simulink model "iqc_lib"  (Simulink 6.0)
settings: Solver=ode45  StartTime=0.0  StopTime=999999  MaxStep=10  RelTol=1e-3  AbsTol=1e-6
libraries: simulink x1
settings Model: Creator=user  LastModifiedBy=MD710
settings DataIOCC: LimitDataPoints=off  SaveOutput=off  SaveTime=off
settings OptimizationCC: BlockReduction=off  BooleanDataType=off  InlineInvariantSignals=off  InitFltsAndDblsToZero=off
settings DebuggingCC: SignalResolutionControl=UseLocalSettings  SolverPrmCheckMsg=none  MultiTaskDSMMsg=warning  MultiTaskCondExecSysMsg=none  FcnCallInpInsideContextMsg=Use local settings  StrictBusMsg=None  SFUnexpectedBacktrackingDiag=warning  SFNoUnconditionalDefaultTransitionDiag=warning
settings HardwareCC: TargetHWDeviceType=32-bit Generic
settings RTWCC: IncludeERTFirstTime=on
settings CodeAppCC: CustomSymbolStrType=$N$R$M

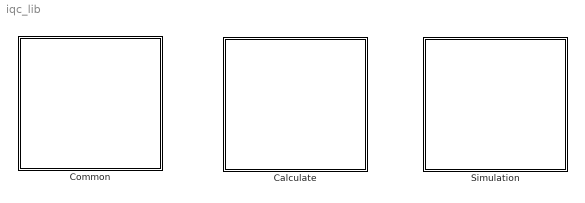
== system iqc_lib ==
  Calculate : Subsystem
      mask Display: disp('Calculate')
  Common : Subsystem
      mask Display: disp('Common')
  Simulation : Subsystem
      mask Display: disp('Simulation')

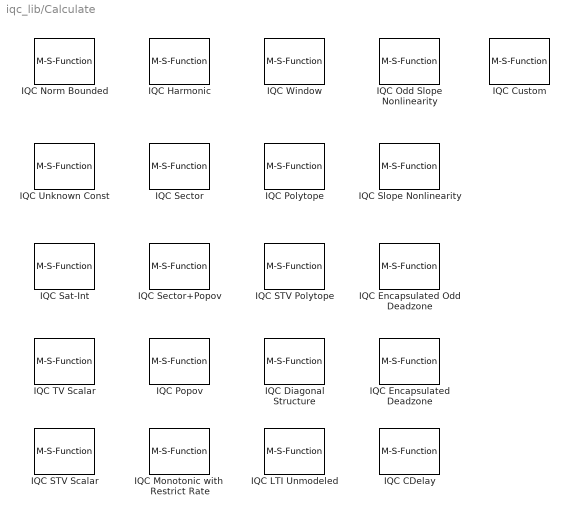
== system iqc_lib/Calculate ==
  IQC CDelay : M-S-Function  MFile=ext_iqc_cdelay  Parameters=max_tim,pole,out_var  mask(IQC cdelay(ver:0.1)){max_tim=1, pole=[], out_var=''}
      mask prompts: max_tim "Maximum Time Delay:(Default: 1)"; pole "Pole:(Default: [])"; out_var "Output Variable:(Default: empty)"
      mask help:
      | Example: [w,X,x]=iqc_cdelay(v,T,a)
      | Maximum Time Delay:
      |         T
      | Pole:
      |        [a]
      | Output Variable:
      |      {'X','x'}
      mask Help: eval('doc iqc_cdelay')
      mask Display: disp('\fontsize{16}e^{-ds}-1', 'texmode','on')
  IQC Custom : M-S-Function  MFile=ext_iqc_custom  Parameters=out_dim,list_iqc_rel  mask(IQC Custom(ver:0.1)){out_dim=-1, list_iqc_rel='out==iqc_popov_vect(in,0)|out==iqc_tvscalar(in,1)'}
      mask prompts: out_dim "Output Signal Dimensions:(Default: -1)"; list_iqc_rel "List of IQC Relationships:"
      mask Display: disp('Custom')
  IQC Diagonal Structure : M-S-Function  MFile=ext_iqc_diag  Parameters=out_var  mask(IQC Diagonal Structure(ver:0.1)){out_var=''}
      mask prompts: out_var "Output Variable:(Default: empty)"
      mask help:
      | Example: [w,X]=iqc_diag(v)
      | Output Variable:
      |             {'X'}
      mask Help: eval('doc iqc_diag')
      mask Display: plot(0,0,100,100,[20,7,7,20],[5,5,94,94],[22,33,11,22],[90,66,66,90],[43,55,32,43],[61,36,36,62],[62,63,62,61,62],[31,29,27,29,31],[71,72,71,70,71],[17,15,13,15,17],[78,90,90,79],[94,94,5,5])
  IQC Encapsulated Deadzone : M-S-Function  MFile=ext_iqc_dzn_e  Parameters=pole,def_num_h,slo_bou,out_var  mask(IQC Encapsulated Deadzone(ver:0.1)){pole=[1], def_num_h=0, slo_bou=1, out_var=''}
      mask prompts: pole "Pole:(Default: [1])"; def_num_h "Defines Number of Terms in Expansion for H:(Default: 0)"; slo_bou "Slope Bound for The Encapsulated Nonlinearity:(Default: 1)"; out_var "Output Variable:(Default: empty)"
      mask help:
      | Example: [w,h_0,H,F,x]=iqc_dzn_e(v,a,N,kdzn)
      | Pole:
      |       [a]
      | Defines Number of Terms in Expansion for H:
      |        N
      | Slope Bound for The Encapsulated Nonlinearity:
      |      kdzn
      | Output Variable:
      |    {'h_0','H','F','x'}
      mask Help: eval('doc iqc_dzn_e')
      mask Display: plot(0,0,100,100,[60,30,30,60,60],[90,90,60,60,90],[30,30,60,60,30],[40,10,10,40,40],[30,10,10,3,30],[25,25,76,76,76],[80,80,60],[72,25,25],[60,77],[76,76],[82,80,77,80,82,98],[76,72,76,80,76,76],[58,50,40,32],[88,76,76,63],[42,45,45,50],[15,17,34,36])
  IQC Encapsulated Odd Deadzone : M-S-Function  MFile=ext_iqc_dzn_e_odd  Parameters=pole,def_num_h,slo_bou,out_var  mask(IQC Encapsulated Odd Deadzone(ver:0.1)){pole=[1], def_num_h=0, slo_bou=1, out_var=''}
      mask prompts: pole "Pole:(Default: [1])"; def_num_h "Defines Number of Terms in Expansion for H:(Default: 0)"; slo_bou "Slope Bound for The Encapsulated Nonlinearity:(Default: 1)"; out_var "Output Variable:(Default: empty)"
      mask help:
      | Example: [w,h_0,H,F,xp,xm]=iqc_dzn_e_odd(v,a,N,kdzn)
      | Pole:
      |         [a]
      | Defines Number of Terms in Expansion for H:
      |          N
      | Slope Bound for The Encapsulated Nonlinearity:
      |         kdzn
      | Output Variable:
      |     {'h_0','H','F','xp','xm'}
      mask Help: eval('doc iqc_dzn_e_odd')
      mask Display: plot(0,0,100,100,[60,30,30,60,60],[90,90,60,60,90],[30,30,60,60,30],[40,10,10,40,40],[30,10,10,3,30],[25,25,76,76,76],[80,80,60],[72,25,25],[60,77],[76,76],[82,80,77,80,82,98],[76,72,76,80,76,76],[58,50,40,32],[88,76,76,63],[42,45,45,50],[15,17,34,36])
  IQC Harmonic : M-S-Function  MFile=ext_iqc_harmonic  Parameters=del_fre,pole,out_var  mask(IQC Harmonic(ver:0.1)){del_fre=1, pole=[1], out_var=''}
      mask prompts: del_fre "Delta Frequency:(Default: 1)"; pole "Pole:(Default: [1])"; out_var "Output Variable:(Default: empty)"
      mask help:
      | Example: [w,P,Q,X]=iqc_harmonic(v,w0,a)
      | Delta Frequency:
      |               w0
      | Pole:
      |               [a]
      | Output Variable:
      |               {'P','Q','X'}
      mask Help: eval('doc iqc_harmonic')
      mask Display: plot(1:0.1:15,cos(1:0.1:15))
  IQC LTI Unmodeled : M-S-Function  MFile=ext_iqc_ltiunmod  Parameters=pole,out_dim,upp_bou,out_var  mask(IQC LTI Unmodeled(ver:0.1)){pole=1, out_dim=-1, upp_bou=1, out_var=''}
      mask prompts: pole "Pole:(Default: [1])"; out_dim "The Dimension of The Output Signal:(Default: -1)"; upp_bou "Upper Bound of The H-inf norm of delta:(Default: 1)"; out_var "Output Variable:(Default: empty)"
      mask help:
      | Example: [w,X]=iqc_ltiunmod(v,a,n,g)
      | Pole:
      |      [a]
      | The Dimension of The Output Signal:
      |       n
      | Upper Bound of The H-inf norm of delta:
      |       g
      | Output Variable:
      |      {'X'}
      mask Help: eval('doc iqc_ltiunmod')
      mask Display:
      | disp('\fontsize{16}\Delta(S)', 'texmode','on');
      | % plot(0,0,100,100,[81,85,86,85,81],[19,34,44,56,72],[54,57,62,71,74,75,74,68,60,55,53,55,60,67,74],[32,27,25,25,28,34,41,48,51,53,59,66,69,69,66],[45,43,42,43,45],[20,37,46,57,72],[25,10,36,25],[71,24,24,72])
  IQC Monotonic with  Restrict Rate : M-S-Function  MFile=ext_iqc_monotonic  Parameters=pole,int_dd,ope,out_var  mask(IQC Monotonic with Restrict Rate(ver:0.1)){pole=[1], ope=0 (shut off the Popov's IQC), int_dd=1, out_var=''}
      mask prompts: pole "Pole:(Default: [1])"; ope "Operator:(Default: 0)"; int_dd "Interval of d(delta)/dt:(Default: 1)"; out_var "Output Variable:(Default: empty)"
      mask help:
      | Example: [w,xa,xb,xc,xd,xpop]=iqc_monotonic(v,a,op,k)
      | Pole:
      |          [a]
      | Operator:
      |          [op]
      | Interval of d(delta)/dt:
      |          [k]
      | Output Variable:
      |          {'xa','xb','xc','xd','xpop'}
      mask Help: eval('doc iqc_monotonic')
      mask StyleString: edit,popup(0 (shut off the Popov's IQC)|1 (turn on the Popov's IQC)),edit,edit
      mask Display: plot(0,0,100,100,[99,-0],[50,50],[50,50],[-0,100],[10,90],[0,100],[99,95,88,82,75,70,67,60,55,50],[76,76,75,74,72,70,68,62,56,50],[1,5,9,16,22,29,34,40,45,50],[20,21,22,24,26,29,32,38,44,50])
  IQC Norm Bounded : M-S-Function  MFile=ext_iqc_ltvnorm  Parameters=out_dim,max_amp,out_var  mask(IQC Norm Bounded(ver:0.1)){out_dim=1, max_amp=1, out_var=''}
      mask prompts: out_dim "The Dimension of the Output Signal:(Default: 1)"; max_amp "Maximal Amplification Ratio:(Default: 1)"; out_var "Output Variable:(Default: Empty)"
      mask help:
      | Example: [w,X]=iqc_ltvnorm(v,n,g)
      | The Dimemsion of the Output Signal:
      |            n
      | Maximal Amplification Ration:
      |            g
      | Output Variable:
      |            {'X'}
      mask Help: eval('doc iqc_ltvnorm')
      mask Display: disp('\fontsize{16}||\Delta|| < k', 'texmode','on')
  IQC Odd Slope Nonlinearity : M-S-Function  MFile=ext_iqc_slope_odd  Parameters=pole,len_def_h,low_bou,upp_bou,out_var  mask(IQC Odd Slope Nonlinearity(ver:0.1)){pole=[1], len_def_h=0, low_bou=0, upp_bou=1, out_var=''}
      mask prompts: pole "Pole:(Default: [1])"; len_def_h "Length of The Expansion that Defines H:(Default: 0)"; low_bou "Lower Bound on Slope:(Default: 0)"; upp_bou "Upper Bound on Slope:(Default: 1)"; out_var "Output Variable:(Default: empty)"
      mask help:
      | Example: [w,h0,H,xp,xm]=iqc_slope_odd(v,a,N,alpha,beta)
      | Pole:
      |          [a]
      | Length of The Expansion that Defines H:
      |           N
      | Lower Bound on Slope:
      |         alpha
      | Upper Bound on Slope:
      |         beta
      | Output Variable:
      |    {'h0','H','xp','xm'}
      mask Help: eval('doc iqc_slope_odd')
      mask Display: plot(0,0,100,100,[96,2],[50,50],[50,50],[95,4],[97,80,60,40,20,4],[90,90,71,30,10,10],[81,84,60,75,60],[72,71,71,99,71],[81,84],[69,71],[73,75],[97,99],[75,75,75],[96,99,99])
  IQC Polytope : M-S-Function  MFile=ext_iqc_polytope  Parameters=arr_pol,out_var  mask(IQC Polytope(ver:0.1)){arr_pol={''}, out_var=''}
      mask prompts: arr_pol "A Cell Array Containing The Vertices of The Polytope:"; out_var "Output Variable:(Default: empty)"
      mask help:
      | Example: [w,X,Y,Z]=iqc_polytope(v,C)
      | A Cell Array Containing The Vertices of The Polytope:
      |                    C
      | Output Variable:
      |              {'X','Y','Z'}
      mask Help: eval('doc iqc_polytope')
      mask Display: plot(0,0,100,100,[33,15,33,67,84,67,33],[80,50,20,20,50,80,80])
  IQC Popov : M-S-Function  MFile=ext_iqc_popov_vect  Parameters=sign_par,out_var  mask(IQC Popov(ver:0.1)){sign_par='0', out_var=''}
      mask prompts: sign_par "Sign of The Popov Parameter:(Default: '0')"; out_var "Output Variable:(Default: empty)"
      mask help:
      | Example: [w,Lambda]=iqc_popov_vect(v,'+')
      | Sign of The Popov Parameter:
      |                     '+'
      | Output Variable:
      |                  {'Lambda'}
      mask Help: eval('doc iqc_popov_vect')
      mask StyleString: popup('0'|'+'|'-'),edit
      mask Display: disp('Popov')
  IQC STV Polytope : M-S-Function  MFile=ext_iqc_polytope_stvp  Parameters=arr_del,arr_ddel,str_mat,out_var  mask(IQC STV Polytope(ver:0.1)){arr_del={''}, arr_ddel={''}, str_mat=[], out_var=''}
      mask prompts: arr_del "Cell Array for delta:"; arr_ddel "Cell Array for d(delta)/dt:"; str_mat "LMI-Lab Structure Matrix:"; out_var "Output Variable:(Default: empty)"
      mask help:
      | Example: [w,X,Y,Z,Lambda]=iqc_polytope_stvp(v,C1,C2,Lambdastruc);
      | Cell Array for delta:
      |              C1
      | Cell Array for d(delta)/dt
      |              C2
      | LMI-Lab Structure Matrix:
      |          Lambdastruc
      | Output Variable:
      |        {'X','Y','Z','Lambda'}
      mask Help: eval('doc iqc_polytope_stvp')
      mask Display: disp('STV\nPolytopic')
  IQC STV Scalar : M-S-Function  MFile=ext_iqc_slowtv  Parameters=upp_bou_dd,pole,upp_bou_d,out_var  mask(IQC STV Scalar(ver:0.1)){upp_bou_dd=1, pole=[1], upp_bou_d=1, out_var=''}
      mask prompts: upp_bou_dd "Upper Bound of The L-inf norm of d(delta)/dt:(Default: 1)"; pole "Pole:(Default [1])"; upp_bou_d "Upper Bound of The L-inf norm of delta:(Default: 1)"; out_var "Output Variable:(Default: empty)"
      mask help:
      | Example: [w,K1,M1,K2,M2]=iqc_slowtv(v,d,a,D)
      | Upper Bound of The L-inf norm of d(delta)/dt:
      |                   d
      | Pole:
      |                  [a]
      | Upper Bound of The L-inf norm of (delta):
      |                   D
      | Output Variable:
      |                  {'K1','M1','K2','M2'}
      mask Help: eval('doc iqc_slowtv')
      mask Display: disp('\fontsize{16}|D^\prime| < k', 'texmode','on')
  IQC Sat-Int : M-S-Function  MFile=ext_iqc_ratelimiter  Parameters=pole,k,out_var  mask(IQC Sat-Int(ver:0.1)){pole=[1,1], k=1, out_var=''}
      mask prompts: pole "Pole:(Default: [1,1])"; k "d(sat(0))/dt Value:(Default: 1)"; out_var "Output Variable:(Default: empty)"
      mask help:
      | Example: [w,M]=iqc_ratelimiter(v,a,k)
      | Pole:
      |     [a]
      | d(sat(0))/dt Value:
      |      k
      | Output Variable:
      |     {'M'}
      mask Help: eval('doc iqc_ratelimiter')
      mask Display: plot(0,0,100,100,[18,45,45,18,18],[60,60,26,26,60],[62,82,82,62,62],[60,60,26,26,60],[62,0],[44,44],[79,65],[44,44],[71,71],[46,57],[68,69,72,74,73,71,69,68,69,72,74],[31,29,29,31,34,35,36,38,40,40,39],[31,31],[26,60],[45,38,24],[55,55,33],[24,18],[33,33],[99,82],[44,44],[10,12,8,10,10,90,90],[44,51,51,44,80,80,44],[7,2],[55,55])
  IQC Sector : M-S-Function  MFile=ext_iqc_sector  Parameters=low_sec,upp_sec,out_var  mask(IQC Sector(ver:0.1)){low_sec=0, upp_sec=1, out_var=''}
      mask prompts: low_sec "Lower Sector Bound:(Default: 0)"; upp_sec "Upper Sector Bound:(Default: 1)"; out_var "Output Variable:(Default: empty)"
      mask help:
      | Example: [w,X]=iqc_sector(v,alpha,beta)
      | Lower Sector Bound:
      |              alpha
      | Upper Sector Bound:
      |              beta
      | Output Variable:
      |              {'X'}
      mask Help: eval('doc iqc_sector')
      mask Display: plot(0,0,100,100,[100,-0],[54,54],[50,50],[0,100],[66,32],[100,0],[-0,100],[37,71],[20,-0],[0,32],[33,13],[5,41],[40,28],[24,46],[47,42],[44,51],[65,57],[60,73],[78,63],[64,90],[95,77],[69,100],[91,85,82,78,77,75,74,66,61,56,54,50,48,45,43,42,40,38,35,31,27,24,21,17,14,11,10,8,7],[96,96,93,90,82,76,71,66,66,63,60,54,51,49,46,42,38,34,32,32,32,32,32,31,29,27,24,18,13])
  IQC Sector+Popov : M-S-Function  MFile=ext_iqc_popov  Parameters=low_sec,upp_sec,out_var  mask(IQC Sector+Popov(ver:0.1)){low_sec=0, upp_sec=1, out_var=''}
      mask prompts: low_sec "Low Sector Bound:(Default: 0)"; upp_sec "Upper Sector Bound:(Default: 1)"; out_var "Output Variable:(Default: empty)"
      mask help:
      | Example: [w,X,Y]=iqc_popov(v,alpha,beta)
      | Low Sector Bound:
      |                alpha
      | Upper Sector Bound:
      |                beta
      | Output Variable:
      |                {'X','Y'}
      mask Help: eval('doc iqc_popov')
      mask Display: plot(0,0,100,100,[100,-0],[54,54],[50,50],[0,100],[66,32],[100,0],[-0,100],[37,71],[20,-0],[0,32],[33,13],[5,41],[40,28],[24,46],[47,42],[44,51],[65,57],[60,73],[78,63],[64,90],[95,77],[69,100],[91,85,82,78,77,75,74,66,61,56,54,50,48,45,43,42,40,38,35,31,27,24,21,17,14,11,10,8,7],[96,96,93,90,82,76,71,66,66,63,60,54,51,49,46,42,38,34,32,32,32,32,32,31,29,27,24,18,13])
  IQC Slope Nonlinearity : M-S-Function  MFile=ext_iqc_slope  Parameters=pole,len_def_h,low_bou,upp_bou,out_var  mask(IQC Slope Nonlinearity(ver:0.1)){pole=[1], len_def_h=0, low_bou=0, upp_bou=1, out_var=''}
      mask prompts: pole "Pole:(Default: [1])"; len_def_h "Length of The Expansion that Defines H:(Default: 0)"; low_bou "Lower Bound on Slope:(Default: 0)"; upp_bou "Upper Bound on Slope:(Default: 1)"; out_var "Output Variable:(Default: empty)"
      mask help:
      | Example: [w,h0,H,x]=iqc_slope(v,a,N,alpha,beta)
      | Pole:
      |         [a]
      | Length of The Expansion that Defines H:
      |          N
      | Lower Bound on Slope:
      |        alpha
      | Upper Bound on Slope:
      |        beta
      | Output Variable:
      |    {'h0','H','x'}
      mask Help: eval('doc iqc_slope')
      mask Display: plot(0,0,100,100,[95,4],[50,50],[50,50],[95,5],[98,79,60,50,40,20,4],[90,90,80,50,40,30,30],[81,84,60,67,60],[82,80,80,100,80],[80,84],[78,80],[64,67],[98,100],[68,67,67,67,67],[96,100,100,100,100])
  IQC TV Scalar : M-S-Function  MFile=ext_iqc_tvscalar  Parameters=upp_bou,out_var  mask(IQC TV Scalar(ver:0.1)){upp_bou=1, out_var=''}
      mask prompts: upp_bou "Upper Bound of The L-inf norm of delta:(Default: 1)"; out_var "Output Variable:(Default: empty)"
      mask help:
      | Example: [w,X,Y]=iqc_tvscalar(v,D)
      | Upper Bound of The L-inf norm of delta:
      |         [D]
      | Output Variable:
      |         {'X','Y'}
      mask Help: eval('doc iqc_tvscalar')
      mask Display: disp('\fontsize{16}|D(t)| < k', 'texmode','on')
  IQC Unknown Const : M-S-Function  MFile=ext_iqc_ltigain  Parameters=pole,out_var  mask(IQC Unknown Const(ver:0.1)){pole=[1], out_var=''}
      mask prompts: pole "Pole:(Default: [1])"; out_var "Output Variable:(Default: Empty)"
      mask help:
      | Example: [w,P,Q,X,Y,Z]=iqc_ltigain(v,a);
      | Pole:
      |       [a]
      | Output Variable:
      |       {'P','Q','X','Y','Z'}
      mask Help: eval('doc iqc_ltigain')
      mask Display: disp('\fontsize{16}|d| < 1', 'texmode','on')
  IQC Window : M-S-Function  MFile=ext_iqc_window  Parameters=max_del,pole,out_var  mask(IQC Window(ver:0.1)){max_del=1, pole=[], out_var=''}
      mask prompts: max_del "Maximum Time Delay:(Default: 1)"; pole "Pole:(Default: [])"; out_var "Output Variable:(Default: empty)"
      mask help:
      | Example: [w,X,Y]=iqc_window(v,T,a)
      | Maximum Time Delay:
      |            T
      | Pole:
      |           [a]
      | Output Variable:
      |          {'X','Y'}
      mask Help: eval('doc iqc_window')
      mask Display: plot(0,0,100,100,[84,94,4],[27,25,25],[94,84],[25,22],[15,15],[5,97],[12,15],[86,97],[18,15],[86,97],[81,70,70,16,16,6],[26,26,72,72,26,26],[71,71,15],[26,73,73])

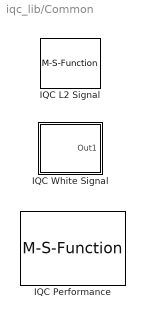
== system iqc_lib/Common ==
  IQC L2 Signal : M-S-Function  MFile=ext_iqc_L2signal  Parameters=sig_size,sam_time,sig_type,tru_time,sig_amp,sig_fre,user_cus  mask(IQC L2 signal(ver:0.1)){sig_size=1, sam_time=0, sig_type=Step, tru_time=10, sig_amp=1, sig_fre=1, user_cus='2*exp(3*t)'}
      mask prompts: sig_size "Signal Dimension:(Default: 1)"; sam_time "Sample Time:(Default: 0)"; sig_type "Signal Type:"; tru_time "Truncation Time:"; sig_amp "Maximum Amplitude:"; sig_fre "Frequency:"; user_cus "Custom:"
      mask help:
      | Important:
      | In IQC procedure step (as commond iqc_gain_tbx, the task is get
      | L2 gain value), regardless of the user to choose which option (ex sine...),
      | here regarded as generalized L2 signal.
      mask StyleString: edit,edit,popup(Step|Square wave|Sine wave|Custom|Random|External),edit,edit,edit,edit
      mask CallbackString: ||iqc_block_cho(gcb,'L2signal_type')||||
      mask TabNameString: Main,Main,Simulation,Simulation,Simulation,Simulation,Simulation
      mask Display: plot(0:0.1:10,[sin(0:0.1:6.2) zeros(1,38)])
  IQC Performance : M-S-Function  MFile=ext_iqc_performance  Parameters=imp_met,save_lin_com,isiqcbode,fre_ran,uselmitool,lmi_par  mask(IQC Performance(ver:0.1)){imp_met=Calculation and Simulation, save_lin_com=off, isiqcbode=off, fre_ran='', uselmitool=lmilab, lmi_par=''}
      mask prompts: imp_met "Implementation Methods"; save_lin_com "Save the Linear File and Command File"; isiqcbode "Display IQC Bode Figure"; fre_ran "Frequency Range:(Default: empty)"; uselmitool "LMI Tool:"; lmi_par "Parameter:(if empty use define)"
      mask help:
      | Important:
      | In IQC toolbox calculate step (as commond iqc_gain_tbx, the task is get
      | L2 gain value), regardless of the user to connect any signal input(Even if
      | not a signal), here regarded as generalized L2 signal.
      |
      | Example 1: setlmioptions('',[0 200 0 0 777])
      | the block parameter is
      | LMI Tool: lmilab
      | Parameter:
      |        [0 200 0 0 777]
      |
      | Example 2: setlmioptions('yalmip','solver','sdpt3','verbose',1)
      | the block parameter is
      | LMI Tool: yalmip
      | Parameter:
      |        {'solver',sdpt3','verbose',1}
      mask Help:
      | <a href="matlab:doc abst_init_iqc;">abst_init_iqc</a>
      | <a href="matlab:doc setlmioptions;">setlmioptions</a>
      | <a href="matlab:doc iqc_gain_tbx;">iqc_gain_tbx</a>
      mask StyleString: popup(Calculation and Simulation|Only Calculation|Only Simulation),checkbox,checkbox,edit,popup(lmilab|yalmip),edit
      mask CallbackString: iqc_block_cho(gcb,'performance_imp')||iqc_block_cho(gcb,'performance_bodefre')|||
      mask TabNameString: Main,Main,Main,Main,LMI,LMI
      mask Display: disp('In -> Out \n performance \n L2 gain:\n Unknown');
  IQC White Signal : Subsystem  mask(IQC White Signal(ver:0.1)){sig_size=1, sam_tim=0, ban_whi=10, pole=[1], out_var='', noi_pow=[0.1], seed=[23341]}
      mask prompts: sig_size "Signal Dimension:(Default: 1)"; sam_tim "Sample Time:(Default: 0)"; ban_whi "Bandwidth of White Signal:(Default: 10)"; pole "Pole:(Default: [1])"; out_var "Output Variable:(Default: empty)"; noi_pow "Noise Power:(Default: [0.1])"; seed "Seed:(Default: [23341])"
      mask help:
      | Example: [f,Y,Z]=iqc_white(n,b,a)
      | Bandwidth of White Signal:
      |           b
      | Pole:
      |           a
      | Output Variable:
      |    {'Y','Z'}
      mask init:
      | if any(noi_pow < 0),
      | 	error('The ''Noise power'' must be positive. '),
      | end;
      | if any(sam_tim==-1), 
      | 	error('You should explicitly specify the sample time of the source block. '), 
      | end
      | 
      | r = [0.4326
      |    -1.6656
      |     0.1253
      |     0.2877
      |    -1.1465
      |     1.1909
      |     -1.1892
      |    0.0376
      |     -0.3273
      |     0.1746
      |    -0.1867
      |     0.7258]';
      | t =[1:13;1:13]; 
      | r2 = [r(1),r;r,r(12)];
      mask Help: eval('doc iqc_white')
      mask TabNameString: Main,Main,Calculation,Calculation,Calculation,Simulation,Simulation
      mask Display: plot(t(:),r2(:))

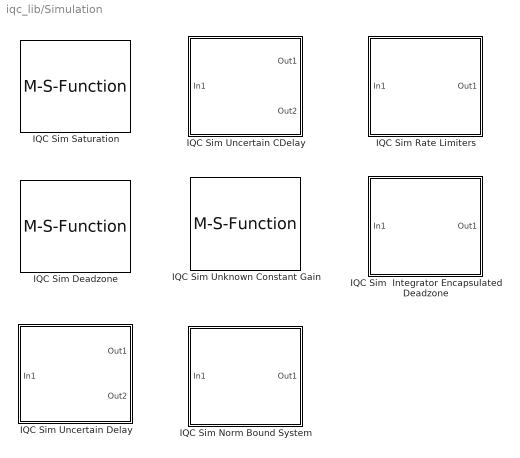
== system iqc_lib/Simulation ==
  IQC Sim Norm Bound System : Subsystem  mask(IQC Sim Norm Bound System(ver:0.1)){sou_sys=Random, num_inp=1, num_out=1, num_sta=1, upp_bou=1, sam_tim=0, cus='1/(s+1)', var_nam='', iqc1=on, iqc1_pole=[1], iqc1_out='', iqc2=off, lis_rel='', swsystemtype=0, A=0, B=0, C=0, D=0, newsam_tim=0}
      mask prompts: sou_sys "Source of the system:(Default: Random)"; num_inp "The Number of Input:(Default: 1)"; num_out "The Number of Output:(Default: 1)"; num_sta "The Number of States:(Default: 1)"; upp_bou "Upper Bound of the Hinf-Norm:(default: 1)"; sam_tim "Sample Time:(Default: 0)"; cus "Custom: (Default: '1/(s+1)' or '1/(z+0.5)')"; var_nam "Variable Name:(Default: empty)"; iqc1 "iqc_ltiunmod(Input,Pole,Number Output,Upper Bound)"; iqc1_pole "Pole:(Default: [1])"; iqc1_out "Output Variable:(Default: empty)"; iqc2 "Custom IQC"; lis_rel "List of IQC Relationships:"
      mask init:
      | swsystemtype=1;
      | A=randn(num_sta);
      | B=randn(num_sta,num_inp);
      | C=randn(num_out,num_sta);
      | D=randn(num_out,num_inp);
      | switch sou_sys
      |     case 1
      |         if sam_tim==0
      |             newsam_tim=1;
      |             A=A-(1+max(real(eig(A))))*eye(num_sta);
      |             G=ss(A,B,C,D);
      |             normG=norm(G,inf);
      |             G=G*upp_bou*rand/normG;
      |         elseif sam_tim>0
      |             newsam_tim=sam_tim;
      |             swsystemtype=2;
      |             A=A-(1+max(real(eig(A))))*eye(num_sta);
      |             G=ss(A,B,C,D);
      |             normG=norm(G,inf);
      |             G=G*upp_bou*rand/normG;
      |             G=c2d(G,sam_tim);
      |         else
      |             error(['sampletime set error'])
      |         end
      |     case 2
      |         s=tf('s');
      |         newsam_tim=1;
      |         if sam_tim>0
      |             newsam_tim=sam_tim;
      |             swsystemtype=2;
      |             z=tf('z',sam_tim);
      |         end
      |         if ischar(cus)
      |             eval(['G=ss(',cus,');']);
      |         else
      |             G=ss(cus);
      |         end
      | end
      | A=G.a;
      | B=G.b;
      | C=G.c;
      | D=G.d;
      mask Help: <a href="matlab:doc iqc_ltiunmod;">iqc_ltiunmod</a>
      mask StyleString: popup(Random|Custom),edit,edit,edit,edit,edit,edit,edit,checkbox,edit,edit,checkbox,edit,edit,edit,edit,edit,edit,edit
      mask CallbackString: iqc_block_cho(gcb,'sim_normboundsys_sou')||||||||iqc_block_cho(gcb,'sim_normboundsys_iqc1')|||iqc_block_cho(gcb,'sim_normboundsys_iqc2')|||||||
      mask TabNameString: Simulation,Simulation,Simulation,Simulation,Simulation,Simulation,Simulation,Simulation,Calculation,Calculation,Calculation,Calculation,Calculation,Simulation,Simulation,Simulation,Simulation,Simulation,Simulation
      mask Display: disp('\fontsize{14}||\Delta|| < k', 'texmode','on')
  IQC Sim Uncertain CDelay : Subsystem  mask(IQC Sim Uncertain CDelay(ver:0.1)){sou_del=Random, max_del=1, num_ran=1, cus=[0], iqc1=on, iqc1_pole=[], iqc1_out='', iqc2=off, lis_rel='', delay_time=0}
      mask prompts: sou_del "Source of the delay:(Default: Random)"; max_del "Maximum Delay:"; num_ran "The Number of Random:(1 or input_dim)"; cus "Custom:"; iqc1 "iqc_cdelay(Input,Maximum Delay,Pole)"; iqc1_pole "Pole:(Default: [])"; iqc1_out "Output Variable:(Default: empty)"; iqc2 "Custom IQC"; lis_rel "List of IQC Relationships:"
      mask init:
      | switch sou_del
      |     case 1
      |         delay_time=max_del*rand(1,num_ran);
      |     case 2
      |         delay_time=reshape(cus,1,length(cus));
      | end
      | % fprintf('The Random Delay Time: %4.3f \n',delay_time);
      mask Help: <a href="matlab:doc iqc_cdelay;">iqc_cdelay</a>
      mask StyleString: popup(Random|Custom),edit,edit,edit,checkbox,edit,edit,checkbox,edit,edit
      mask CallbackString: iqc_block_cho(gcb,'sim_uncertaincdelay_sou')||||iqc_block_cho(gcb,'sim_uncertaincdelay_iqc1')|||iqc_block_cho(gcb,'sim_uncertaincdelay_iqc2')||
      mask TabNameString: Simulation,Simulation,Simulation,Simulation,Calculation,Calculation,Calculation,Calculation,Calculation,Simulation
      mask Display:
      | disp('\fontsize{14}exp(-T*s)-1', 'texmode','on')
      | port_label('input',1,'in');
      | port_label('output',1,'out');
      | port_label('output',2,'T');
  IQC Sim Uncertain Delay : Subsystem  mask(IQC Sim Uncertain Delay(ver:0.1)){sou_del=Custom, max_del=1, num_ran=1, cus=[0.5], iqc1=on, iqc1_pole=[], iqc1_out='', iqc2=off, iqc2_pole=[], iqc2_out='', iqc3=off, lis_rel='', delay_time=0}
      mask prompts: sou_del "Source of the delay:(Default: Random)"; max_del "Maximum Delay:"; num_ran "The Number of Random:(1 or input_dim)"; cus "Custom:"; iqc1 "iqc_delay(Input,Maximum Delay,Pole)"; iqc1_pole "Pole:(Default: [])"; iqc1_out "Output Variable:(Default: empty)"; iqc2 "iqc_delay1(Input,Maximum Delay,Pole)"; iqc2_pole "Pole:(Default: [])"; iqc2_out "Output Variable:(Default: empty)"; iqc3 "Custom IQC"; lis_rel "List of IQC Relationships:"
      mask init:
      | switch sou_del
      |     case 1
      |         delay_time=max_del*rand(1,num_ran);
      |     case 2
      |         delay_time=reshape(cus,1,length(cus));
      | end
      | % fprintf('The Random Delay Time: %4.3f \n',delay_time);
      mask Help:
      | <a href="matlab:doc iqc_delay;">iqc_delay</a>
      | <a href="matlab:doc iqc_delay1;">iqc_delay1</a>
      mask StyleString: popup(Random|Custom),edit,edit,edit,checkbox,edit,edit,checkbox,edit,edit,checkbox,edit,edit
      mask CallbackString: iqc_block_cho(gcb,'sim_uncertaindelay_sou')||||iqc_block_cho(gcb,'sim_uncertaindelay_iqc1')|||iqc_block_cho(gcb,'sim_uncertaindelay_iqc2')|||iqc_block_cho(gcb,'sim_uncertaindelay_iqc3')||
      mask TabNameString: Simulation,Simulation,Simulation,Simulation,Calculation,Calculation,Calculation,Calculation,Calculation,Calculation,Calculation,Calculation,Simulation
      mask Display:
      | disp('\fontsize{14}exp(-T*s)', 'texmode','on')
      | port_label('input',1,'in');
      | port_label('output',1,'out');
      | port_label('output',2,'T');
  IQC Sim Unknown Constant Gain : M-S-Function  MFile=ext_sim_unknown_gain  Parameters=sou_con,num_ran,cus,iqc1,iqc1_pole,iqc1_out,iqc2,iqc2_out,iqc3,iqc3_out,iqc4,lis_rel,rand_cons  mask(IQC Sim Unknown Constant Gain(ver:0.1)){sou_con=Random, num_ran=1, cus=[0], iqc1=on, iqc1_pole=[1], iqc1_out='', iqc2=off, iqc2_out='', iqc3=off, iqc3_out='', iqc4=off, lis_rel='', rand_cons=0}
      mask prompts: sou_con "Source of The Constant Gain:(Default: Random)"; num_ran "The Number of Random:(1 or input_dim)"; cus "Custom:"; iqc1 "iqc_ltigain(Input,Pole)"; iqc1_pole "Pole:(Default: [1])"; iqc1_out "Output Variable:(Default: empty)"; iqc2 "iqc_ltvnorm(Input,length(Input),1)"; iqc2_out "Output Variable:(Default: empty)"; iqc3 "iqc_tvscalar(Input,1)"; iqc3_out "Output Variable:(Default: empty)"; iqc4 "Custom IQC"; lis_rel "List of IQC Relationships:"
      mask init:
      | switch sou_con
      |     case 1
      |         rand_cons=rand(1,num_ran);
      |     case 2
      |         if any(abs(cus)>1)
      |             error('the maximum random constant is 1')
      |         else
      |             rand_cons=reshape(cus,1,length(cus));
      |         end
      | end
      mask Help:
      | <a href="matlab:doc iqc_ltigain;">iqc_ltigain</a>
      | <a href="matlab:doc iqc_ltvnorm;">iqc_ltvnorm</a>
      | <a href="matlab:doc iqc_tvscalar;">iqc_tvscalar</a>
      mask StyleString: popup(Random|Custom),edit,edit,checkbox,edit,edit,checkbox,edit,checkbox,edit,checkbox,edit,edit
      mask CallbackString: iqc_block_cho(gcb,'sim_constantgain_sou')|||iqc_block_cho(gcb,'sim_constantgain_iqc1')|||iqc_block_cho(gcb,'sim_constantgain_iqc2')||iqc_block_cho(gcb,'sim_constantgain_iqc3')||iqc_block_cho(gcb,'sim_constantgain_iqc4')||
      mask TabNameString: Simulation,Simulation,Simulation,Calculation,Calculation,Calculation,Calculation,Calculation,Calculation,Calculation,Calculation,Calculation,Simulation
      mask Display:
      | disp('\fontsize{14}|d| < 1', 'texmode','on');
      | port_label('input',1,'in');
      | port_label('output',1,'out');
      | port_label('output',2,'|d|');
  IQC Sim  Integrator Encapsulated Deadzone : Subsystem  mask(IQC Sim Integrator Encapsulated Deadzone(ver:0.1)){sta_dea=-1, end_dea=1, slo=1, iqc1=on, iqc1_pole=[1], iqc1_def_num_h=0, iqc1_out='', iqc2=off, iqc2_pole=[1], iqc2_def_num_h=0, iqc2_out='', iqc3=off, lis_rel=''}
      mask prompts: sta_dea "Start of Deadzone:"; end_dea "End of Deadzone:"; slo "Slope:"; iqc1 "iqc_dzn_e(Input,Pole,N,Slope)"; iqc1_pole "Pole:(Default: [1])"; iqc1_def_num_h "Defines Number of Terms in Expansion for H:(Default: 0)"; iqc1_out "Output Variable:(Default: empty)"; iqc2 "iqc_dzn_e_odd(Input,Pole,N,Slope)"; iqc2_pole "Pole:(Default: [1])"; iqc2_def_num_h "Defines Number of Terms in Expansion for H:(Default: 0)"; iqc2_out "Output Variable:(Default: empty)"; iqc3 "Custom IQC"; lis_rel "List of IQC Relationships:"
      mask Help:
      | <a href="matlab:doc iqc_dzn_e;">iqc_dzn_e</a>
      | <a href="matlab:doc iqc_dzn_e_odd;">iqc_dzn_e_odd</a>
      mask CallbackString: |||iqc_block_cho(gcb,'sim_intencdeadzone_iqc1')||||iqc_block_cho(gcb,'sim_intencdeadzone_iqc2')||||iqc_block_cho(gcb,'sim_intencdeadzone_iqc3')|
      mask TabNameString: Simulation,Simulation,Simulation,Calculation,Calculation,Calculation,Calculation,Calculation,Calculation,Calculation,Calculation,Calculation,Calculation
      mask Display: plot(0,0,100,100,[60,30,30,60,60],[90,90,60,60,90],[30,30,60,60,30],[40,10,10,40,40],[30,10,10,3,30],[25,25,76,76,76],[80,80,60],[72,25,25],[60,77],[76,76],[82,80,77,80,82,98],[76,72,76,80,76,76],[58,50,40,32],[88,76,76,63],[42,45,45,50],[15,17,34,36])
  IQC Sim Deadzone : M-S-Function  MFile=ext_sim_deadzone  Parameters=sta_dea,end_dea,sam_tim,iqc1,iqc1_pole,iqc1_ope,iqc1_out,iqc2,iqc2_out,iqc3,iqc3_out,iqc4,iqc4_sign,iqc4_out,iqc5,lis_rel  mask(IQC Sim Deadzone(ver:0.2)){sta_dea=-1, end_dea=1, sam_tim=0, iqc1=on, iqc1_pole=[1], iqc1_ope=0 (shut off the Popov's IQC), iqc1_out='', iqc2=off, iqc2_out='', iqc3=off, iqc3_out='', iqc4=off, iqc4_sign='0', iqc4_out='', iqc5=off, lis_rel=''}
      mask prompts: sta_dea "Start of Deadzone:"; end_dea "End of Deadzone:"; sam_tim "Sample Time:"; iqc1 "iqc_monotonic(Input,Pole,Operator,1) (only for scalar input)"; iqc1_pole "Pole:(Default:[1])"; iqc1_ope "Operator:(Default: 0)"; iqc1_out "Output Variable:(Default: empty)"; iqc2 "iqc_sector(Input,0,1) (only for scalar input)"; iqc2_out "Output Variable:(Default: empty)"; iqc3 "iqc_popov(Input,0,1) (only for scalar input)"; iqc3_out "Output Variable:(Default: empty)"; iqc4 "iqc_popov_vect(Input,Sign)"; iqc4_sign "Sign:(Default: '0')"; iqc4_out "Output Variable:(Default: empty)"; iqc5 "Custom IQC"; lis_rel "List of IQC Relationships:"
      mask Help:
      | <a href="matlab:doc iqc_monotonic;">iqc_monotonic</a>
      | <a href="matlab:doc iqc_sector;">iqc_sector</a>
      | <a href="matlab:doc iqc_popov;">iqc_popov</a>
      | <a href="matlab:doc iqc_popov_vect;">iqc_popov_vect</a>
      mask StyleString: edit,edit,edit,checkbox,edit,popup(0 (shut off the Popov's IQC)|1 (turn on the Popov's IQC)),edit,checkbox,edit,checkbox,edit,checkbox,popup('0'|'+'|'-'),edit,checkbox,edit
      mask CallbackString: |||iqc_block_cho(gcb,'sim_deadzone_iqc1')||||iqc_block_cho(gcb,'sim_deadzone_iqc2')||iqc_block_cho(gcb,'sim_deadzone_iqc3')||iqc_block_cho(gcb,'sim_deadzone_iqc4')|||iqc_block_cho(gcb,'sim_deadzone_iqc5')|
      mask TabNameString: Simulation,Simulation,Simulation,Calculation,Calculation,Calculation,Calculation,Calculation,Calculation,Calculation,Calculation,Calculation,Calculation,Calculation,Calculation,Calculation
      mask Display:
      | x=-5:5;
      | for i=1:11
      |     if x(i)>=-2 && x(i)<=2
      |         y(i)=0;
      |     elseif x(i)<-2
      |         y(i)=x(i)+2;
      |     elseif x(i)>2
      |         y(i)=x(i)-2;
      |     end
      | end
      | x1=zeros(1,11);
      | y1=-5:1:5;
      | y2=zeros(1,11);
      | plot(x,y);
      | plot(x1,y1);
      | plot(x,y2);
  IQC Sim Rate Limiters : Subsystem  mask(IQC Sim Rate Limiters(ver:0.1)){upp_lim=1, low_lim=-1, d_sat=1, firstpole=1, iqc1=on, iqc1_pole=[1], iqc1_out='', iqc2=off, lis_rel=''}
      mask prompts: upp_lim "Upper Limit of Saturation:"; low_lim "Lower Limit of Saturation:"; d_sat "Slope of Saturation:(Default: 1)"; firstpole "(s+Pole1) ~ the Pole1:(Default: 1)"; iqc1 "iqc_ratelimiter(Input,[Pole1 Pole],Slope)  (only for scalar input)"; iqc1_pole "Pole:(Default: [1])"; iqc1_out "Output Variable:(Default: empty)"; iqc2 "Custom IQC"; lis_rel "List of IQC Relationships:"
      mask init:
      | if length(firstpole)>1
      |     error('the Pole1 only scalar')
      | end
      | if length(d_sat)>1
      |     error('d(Sat(0))/dt only scalar')
      | end
      mask Help: <a href="matlab:doc iqc_ratelimiter;">iqc_ratelimiter</a>
      mask CallbackString: ||||iqc_block_cho(gcb,'sim_ratelim_iqc1')|||iqc_block_cho(gcb,'sim_ratelim_iqc2')|
      mask TabNameString: Simulation,Simulation,Simulation,Simulation,Calculation,Calculation,Calculation,Calculation,Calculation
      mask Display: plot(0,0,100,100,[18,45,45,18,18],[60,60,26,26,60],[62,82,82,62,62],[60,60,26,26,60],[62,0],[44,44],[79,65],[44,44],[71,71],[46,57],[68,69,72,74,73,71,69,68,69,72,74],[31,29,29,31,34,35,36,38,40,40,39],[31,31],[26,60],[45,38,24],[55,55,33],[24,18],[33,33],[99,82],[44,44],[10,12,8,10,10,90,90],[44,51,51,44,80,80,44],[7,2],[55,55])
  IQC Sim Saturation : M-S-Function  MFile=ext_sim_saturation  Parameters=upp_lim,low_lim,sam_tim,iqc1,iqc1_pole,iqc1_ope,iqc1_out,iqc2,iqc2_out,iqc3,iqc3_out,iqc4,iqc4_sign,iqc4_out,iqc5,lis_rel  mask(IQC Sim Saturation(ver:0.1)){upp_lim=1, low_lim=-1, sam_tim=0, iqc1=on, iqc1_pole=[1], iqc1_ope=0 (shut off the Popov's IQC), iqc1_out='', iqc2=off, iqc2_out='', iqc3=off, iqc3_out='', iqc4=off, iqc4_sign='0', iqc4_out='', iqc5=off, lis_rel=''}
      mask prompts: upp_lim "Upper Limit:"; low_lim "Lower Limit:"; sam_tim "Sample Time:(Default: 0)"; iqc1 "iqc_monotonic(Input,Pole,Operator,1) (only for scalar input)"; iqc1_pole "Pole:(Default:[1])"; iqc1_ope "Operator:(Default: 0)"; iqc1_out "Output Variable:(Default: empty)"; iqc2 "iqc_sector(Input,0,1) (only for scalar input)"; iqc2_out "Output Variable:(Default: empty)"; iqc3 "iqc_popov(Input,0,1) (only for scalar input)"; iqc3_out "Output Variable:(Default: empty)"; iqc4 "iqc_popov_vect(Input,Sign)"; iqc4_sign "Sign:(Default: '0')"; iqc4_out "Output Variable:(Default: empty)"; iqc5 "Custom IQC"; lis_rel "List of IQC Relationships:"
      mask Help:
      | <a href="matlab:doc iqc_monotonic;">iqc_monotonic</a>
      | <a href="matlab:doc iqc_sector;">iqc_sector</a>
      | <a href="matlab:doc iqc_popov;">iqc_popov</a>
      | <a href="matlab:doc iqc_popov_vect;">iqc_popov_vect</a>
      mask StyleString: edit,edit,edit,checkbox,edit,popup(0 (shut off the Popov's IQC)|1 (turn on ther Popov's IQC)),edit,checkbox,edit,checkbox,edit,checkbox,popup('0'|'+'|'-'),edit,checkbox,edit
      mask CallbackString: |||iqc_block_cho(gcb,'sim_saturation_iqc1')||||iqc_block_cho(gcb,'sim_saturation_iqc2')||iqc_block_cho(gcb,'sim_saturation_iqc3')||iqc_block_cho(gcb,'sim_saturation_iqc4')|||iqc_block_cho(gcb,'sim_saturation_iqc5')|
      mask TabNameString: Simulation,Simulation,Simulation,Calculation,Calculation,Calculation,Calculation,Calculation,Calculation,Calculation,Calculation,Calculation,Calculation,Calculation,Calculation,Calculation
      mask Display:
      | x=-10:10;
      | for i=1:21;
      |     if x(i)>=-3 && x(i)<=3;
      |         y(i)=x(i);
      |     elseif x(i)<-3;
      |         y(i)=-3;
      |     elseif x(i)>3;
      |         y(i)=3;
      |     end
      | end
      | x1=zeros(1,11);
      | y1=-5:1:5;
      | y2=zeros(1,21);
      | plot(x,y);
      | plot(x1,y1);
      | plot(x,y2);

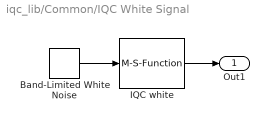
== system iqc_lib/Common/IQC White Signal ==
  Band-Limited White Noise : simulink/Sources/Band-Limited White Noise  Cov=noi_pow  Ts=sam_tim+0.01  seed=seed
  IQC white : M-S-Function  MFile=ext_iqc_white  Parameters=sig_size,ban_whi,pole,out_var,sam_tim
      mask Display: disp('IQC white \n S-function')
  Out1 : Outport
  wires:
  IQC white/1 -> Out1/1
  Band-Limited White Noise/1 -> IQC white/1

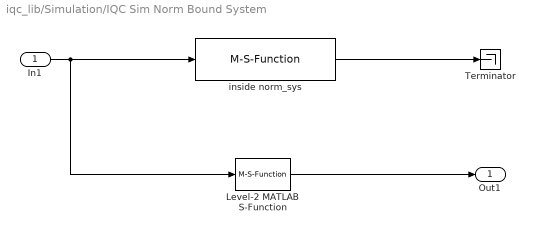
== system iqc_lib/Simulation/IQC Sim Norm Bound System ==
  In1 : Inport
  Level-2 MATLAB S-Function : M-S-Function  MFile=IQCSimSystem  Parameters=A,B,C,D,sam_tim
  Terminator : Terminator
  inside norm_sys : M-S-Function  MFile=ext_sim_normboundsystem  Parameters=sou_sys,num_inp,num_out,num_sta,upp_bou,sam_tim,cus,var_nam,iqc1,iqc1_pole,iqc1_out,iqc2,lis_rel,swsystemtype,A,B,C,D,
  Out1 : Outport
  wires:
  inside norm_sys/1 -> Terminator/1
  In1/1 -> Level-2 MATLAB S-Function/1, inside norm_sys/1
  Level-2 MATLAB S-Function/1 -> Out1/1

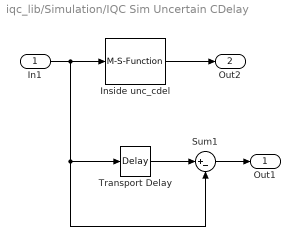
== system iqc_lib/Simulation/IQC Sim Uncertain CDelay ==
  In1 : Inport
  Inside unc_cdel : M-S-Function  MFile=ext_sim_uncertain_cdelay  Parameters=sou_del,max_del,num_ran,cus,iqc1,iqc1_pole,iqc1_out,iqc2,lis_rel,delay_time
  Sum1 : Sum  Inputs=|+-
  Transport Delay : TransportDelay  DelayTime=delay_time
  Out1 : Outport
  Out2 : Outport  Port=2
  wires:
  Inside unc_cdel/1 -> Out2/1
  Transport Delay/1 -> Sum1/1
  In1/1 -> Inside unc_cdel/1, Transport Delay/1, Sum1/2
  Sum1/1 -> Out1/1

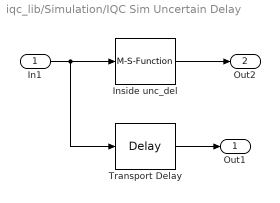
== system iqc_lib/Simulation/IQC Sim Uncertain Delay ==
  In1 : Inport
  Inside unc_del : M-S-Function  MFile=ext_sim_uncertain_delay  Parameters=sou_del,max_del,num_ran,cus,iqc1,iqc1_pole,iqc1_out,iqc2,iqc2_pole,iqc2_out,iqc3,lis_rel,delay_time
  Transport Delay : TransportDelay  DelayTime=delay_time
  Out1 : Outport
  Out2 : Outport  Port=2
  wires:
  In1/1 -> Inside unc_del/1, Transport Delay/1
  Transport Delay/1 -> Out1/1
  Inside unc_del/1 -> Out2/1

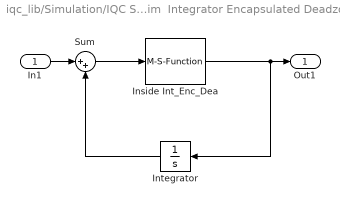
== system iqc_lib/Simulation/IQC Sim  Integrator Encapsulated Deadzone ==
  In1 : Inport
  Inside Int_Enc_Dea : M-S-Function  MFile=ext_sim_intenc_deadzone  Parameters=sta_dea,end_dea,slo,iqc1,iqc1_pole,iqc1_def_num_h,iqc1_out,iqc2,iqc2_pole,iqc2_def_num_h,iqc2_out,iqc3,lis_rel
  Integrator : Integrator  Orientation=left
  Sum : Sum  Inputs=|++
  Out1 : Outport
  wires:
  Inside Int_Enc_Dea/1 -> Out1/1, Integrator/1
  Sum/1 -> Inside Int_Enc_Dea/1
  Integrator/1 -> Sum/2
  In1/1 -> Sum/1

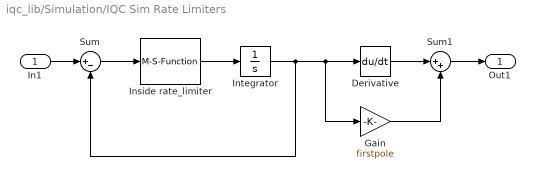
== system iqc_lib/Simulation/IQC Sim Rate Limiters ==
  In1 : Inport
  Derivative : Derivative
  Gain : Gain  Gain=firstpole
  Inside rate_limiter : M-S-Function  MFile=ext_sim_rate_limiter  Parameters=upp_lim,low_lim,d_sat,firstpole,iqc1,iqc1_pole,iqc1_out,iqc2,lis_rel
  Integrator : Integrator
  Sum : Sum  Inputs=|+-
  Sum1 : Sum  Inputs=|++
  Out1 : Outport
  wires:
  Gain/1 -> Sum1/2
  Derivative/1 -> Sum1/1
  Inside rate_limiter/1 -> Integrator/1
  Integrator/1 -> Gain/1, Derivative/1, Sum/2
  Sum/1 -> Inside rate_limiter/1
  Sum1/1 -> Out1/1
  In1/1 -> Sum/1
